simulink model "SPSAS"  (Simulink 7.5)
settings: Solver=ode45  StartTime=0.0  StopTime=2.0  RelTol=1e-3
values from neighbouring files (symbols this model uses):
  Asp = [-1.47961 -49.4425;1 -1.16668]    [Short_Period_SAS.m]
  Bsp = [-22.4739;-0.121741]    [Short_Period_SAS.m]
  Csp = eye(2)    [Short_Period_SAS.m]
  Dsp = zeros(2,1)    [Short_Period_SAS.m]
settings Model: Creator=Compaq_Propietario  LastModifiedBy=Compaq_Propietario
settings DebuggingCC: SolverPrmCheckMsg=none

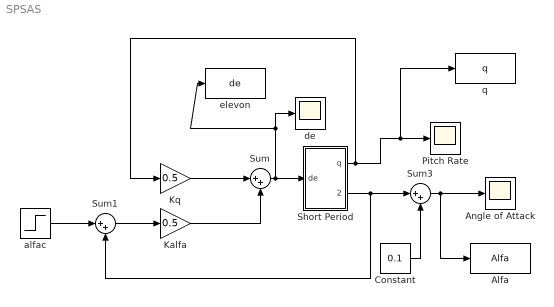
== system SPSAS ==
  Alfa : ToWorkspace  VariableName=Alfa  SampleTime=-1  SaveFormat=Array
  Angle of Attack : Scope
  Constant : Constant  Value=0.1  OutDataType=fixdt(1, 16)  OutScaling=2^0
  Kalfa : Gain  Gain=0.5  ParameterDataType=fixdt(1, 16)  ParameterScaling=2^0  OutDataType=fixdt(1, 16)  OutScaling=2^0
  Kq : Gain  Gain=0.5  ParameterDataType=fixdt(1, 16)  ParameterScaling=2^0  OutDataType=fixdt(1, 16)  OutScaling=2^0
  Pitch Rate : Scope
  Short Period : Subsystem
  Sum : Sum  Inputs=|++  OutDataType=fixdt(1, 16)  OutScaling=2^0
  Sum1 : Sum  Inputs=|++  OutDataType=fixdt(1, 16)  OutScaling=2^0
  Sum3 : Sum  Inputs=|++  OutDataType=fixdt(1, 16)  OutScaling=2^0
  alfac : Step  Time=0  After=0.1  SampleTime=0
  de : Scope
      settings: SaveName=ScopeData2
  elevon : ToWorkspace  VariableName=de  SampleTime=-1  SaveFormat=Array
  q : ToWorkspace  VariableName=q  SampleTime=-1  SaveFormat=Array
  wires:
  Sum/1 -> Short Period/1(de), de/1, elevon/1
  Short Period/2(alfa) -> Sum3/1, Sum1/2
  Sum1/1 -> Kalfa/1
  Short Period/1(q) -> Kq/1, Pitch Rate/1, q/1
  alfac/1 -> Sum1/1
  Constant/1 -> Sum3/2
  Sum3/1 -> Angle of Attack/1, Alfa/1
  Kq/1 -> Sum/1
  Kalfa/1 -> Sum/2

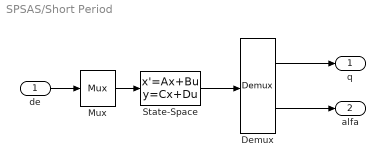
== system SPSAS/Short Period ==
  de : Inport  OutDataType=sfix(16)  OutScaling=2^0
  Demux : Demux  Outputs=2
  Mux : Mux  Inputs=1
  State-Space : StateSpace  A=Asp  B=Bsp  C=Csp  D=Dsp
  q : Outport  OutDataType=sfix(16)  OutScaling=2^0  InitialOutput=0
  alfa : Outport  Port=2  OutDataType=sfix(16)  OutScaling=2^0  InitialOutput=0
  wires:
  Mux/1 -> State-Space/1
  de/1 -> Mux/1
  Demux/1 -> q/1
  Demux/2 -> alfa/1
  State-Space/1 -> Demux/1
